simulink model "demd_dcMotor_separatelyExcit_f1"  (R2021a)
settings: Solver=VariableStepAuto  StartTime=0.0  StopTime=800  RelTol=1e-3
values from neighbouring files (symbols this model uses):
  B = (p_acc/3)/omega_n^2    (= 0.976675486798)    [demd_e2_dcMotor_separatelyExcited.m]
  C1 = 16.7/314    (= 0.0531847133758)    [demd_e2_dcMotor_separatelyExcited.m]
  C3 = 314/60    (= 5.23333333333)    [demd_e2_dcMotor_separatelyExcited.m]
  En = Ve/Ie    (= 120)    [demd_e2_dcMotor_separatelyExcited.m]
  Ie = 1    [demd_e2_dcMotor_separatelyExcited.m]
  J = M*v_max^2/omega_n^2    (= 73.2506615098)    [demd_e2_dcMotor_separatelyExcited.m]
  K = T_n/(I_n*Ie)    (= 1.71974522293)    [demd_e2_dcMotor_separatelyExcited.m]
  ki_curr = wia*Ra    (= 0.00168230769231)    [demd_e2_dcMotor_separatelyExcited.m]
  ki_exc = wie*Re    (= 24)    [demd_e2_dcMotor_separatelyExcited.m]
  ki_speed = ws*B    (= 1.9533509736)    [demd_e2_dcMotor_separatelyExcited.m]
  kp_curr = wia*La    (= 1.68230769231e-05)    [demd_e2_dcMotor_separatelyExcited.m]
  kp_exc = wie*Le    (= 24)    [demd_e2_dcMotor_separatelyExcited.m]
  kp_speed = ws*J    (= 146.50132302)    [demd_e2_dcMotor_separatelyExcited.m]
  La = Ra*tau_a    (= 0.000841153846154)    [demd_e2_dcMotor_separatelyExcited.m]
  Le = Re*tau_e    (= 120)    [demd_e2_dcMotor_separatelyExcited.m]
  Ra = (1-eta)*v_n/I_n    (= 0.0841153846154)    [demd_e2_dcMotor_separatelyExcited.m]
  Re = Ve/Ie    (= 120)    [demd_e2_dcMotor_separatelyExcited.m]
  T_n = p_tot/omega_n    (= 1226.70441142)    [demd_e2_dcMotor_separatelyExcited.m]
  v_n = 600    [demd_e2_dcMotor_separatelyExcited.m]
  Ve = 120    [demd_e2_dcMotor_separatelyExcited.m]
undefined symbols (not defined in the file or in its folder): Antiwindup
libraries: pid_lib x5, simulink x4
settings Model: Creator=mluser  LastModifiedBy=mluser
settings SolverCC: ZeroCrossAlgorithm=Adaptive  AlgebraicLoopSolver=TrustRegion
settings DebuggingCC: IgnoredZcDiagnostic=none

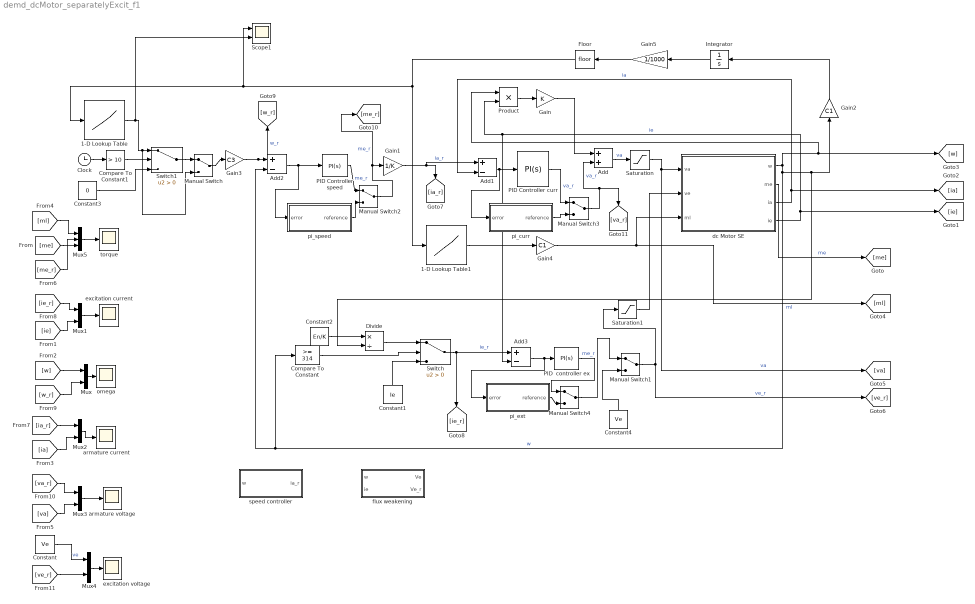
== system demd_dcMotor_separatelyExcit_f1 ==
  1-D Lookup Table : Lookup_n-D  NumberOfTableDimensions=1  BreakpointsForDimension1=[0 1 3 4 6 8 9 10]  Table=[35 60 60 75 60 60 35 0]  InterpMethod=Flat  InternalRulePriority=Speed  RndMeth=Simplest  InputSameDT=on
  1-D Lookup Table1 : Lookup_n-D  NumberOfTableDimensions=1  BreakpointsForDimension1=[0 1 3 4 6 8 9 10]  Table=[0 0 26000*9.81*sin(atan(5/100)) 0 0 26000*9.81*sin(atan(-5/100)) 0 0]  InterpMethod=Flat  InternalRulePriority=Speed  RndMeth=Simplest  InputSameDT=on
  Add : Sum
  Add1 : Sum  Inputs=+-
  Add2 : Sum  Inputs=+-
  Add3 : Sum  Inputs=+-
  Clock : Clock
  Compare To Constant : simulink/Logic and Bit Operations/Compare To Constant  relop=>=  const=314  OutDataTypeStr=boolean
  Compare To Constant1 : simulink/Logic and Bit Operations/Compare To Constant  relop=>  const=10  OutDataTypeStr=boolean
  Constant : Constant  Value=Ve
  Constant1 : Constant  Value=Ie
  Constant2 : Constant  Value=En/K
  Constant3 : Constant  Value=0
  Constant4 : Constant  Value=Ve
  Divide : Product  Inputs=*/
  Floor : Rounding
  Gain : Gain  Gain=K
  Gain1 : Gain  Gain=1/K
  Gain2 : Gain  Gain=C1
  Gain3 : Gain  Gain=C3
  Gain4 : Gain  Gain=C1
  Gain5 : Gain  Gain=1/1000
  Integrator : Integrator
  Manual Switch{,1..4} (5 alike) : ManualSwitch
  Mux{,1..4} (5 alike) : Mux  Inputs=2
  Mux5 : Mux  Inputs=3
  PID  controller ex : pid_lib/PID Controller  Controller=PI  Form=Parallel  TimeDomain=Continuous-time  UseExternalTs=off  SampleTime=-1  IntegratorMethod=Forward Euler  FilterMethod=Forward Euler  ControllerParametersSource=internal  P=kp_exc  I=ki_exc  D=0  UseFilter=on  N=100  TunerSelectOption=Transfer Function Based (PID Tuner App)  InitialConditionSource=internal  InitialConditionForIntegrator=0  InitialConditionForFilter=0  DifferentiatorICPrevScaledInput=0  ExternalReset=none  TrackingMode=off  Kt=1  LimitOutput=on  SatLimitsSource=internal  UpperSaturationLimit=Ve+Ve*0.3  LowerSaturationLimit=-1.3*Ve  LinearizeAsGain=on  AntiWindupMode=clamping  Kb=1  POutMin=[]  POutMax=[]  IOutMin=[]  IOutMax=[]  DOutMin=[]  DOutMax=[]  NOutMin=[]  NOutMax=[]  SumOutMin=[]  SumOutMax=[]  SaturationOutMin=[]  SaturationOutMax=[]  PParamMin=[]  PParamMax=[]  IParamMin=[]  IParamMax=[]  DParamMin=[]  DParamMax=[]  NParamMin=[]  NParamMax=[]  KbParamMin=[]  KbParamMax=[]  KtParamMin=[]  KtParamMax=[]  KbOutMin=[]  KbOutMax=[]  KtOutMin=[]  KtOutMax=[]  IntegratorOutMin=[]  IntegratorOutMax=[]  FilterOutMin=[]  FilterOutMax=[]  SumI1OutMin=[]  SumI1OutMax=[]  SumI2OutMin=[]  SumI2OutMax=[]  SumI3OutMin=[]  SumI3OutMax=[]  SumI4OutMin=[]  SumI4OutMax=[]  SumDOutMin=[]  SumDOutMax=[]  DifferentiatorOutMin=[]  DifferentiatorOutMax=[]  FilterDiffOutCoefMin=[]  FilterDiffOutCoefMax=[]  ReciprocalOutMin=[]  ReciprocalOutMax=[]  SumDenOutMin=[]  SumDenOutMax=[]  SumNumOutMin=[]  SumNumOutMax=[]  DivideOutMin=[]  DivideOutMax=[]  UdiffTsProdOutMin=[]  UdiffTsProdOutMax=[]  NTsProdOutMin=[]  NTsProdOutMax=[]  UintegralTsProdOutMin=[]  UintegralTsProdOutMax=[]  UngainTsProdOutMin=[]  UngainTsProdOutMax=[]  IntegratorContinuousStateAttributes=''  IntegratorStateMustResolveToSignalObject=off  IntegratorRTWStateStorageClass=Auto  FilterContinuousStateAttributes=''  FilterStateMustResolveToSignalObject=off  FilterRTWStateStorageClass=Auto  ParallelPVariant=InternalParameters  IdealPVariant=Disabled  IVariant=InternalParameters  DVariant=Disabled  IntegratorVariant=Continuous  SatVariant=Enabled  AWVariant=ContClampingParallel  PCopyVariant=Disabled  TRVariant=Disabled  FdbkBlocksVariant=Forward  IdealPFdbkVariant=Disabled  SatFdbkVariant=Disabled  DerivativeFilterVariant=Disabled  NVariant=Disabled  NCopyVariant=Disabled_SignalSpec  FilterICVariant=Disabled  IntegratorICVariant=InternalICs  ExternalResetVariant=Disabled  TRSumVariant=Passthrough  SumFdbkVariant=Disabled  SumVariant=Sum_PI  TsampFilterVariant=InternalTs  TsampNgainVariant=Passthrough  TsampIntegralVariant=Passthrough  ExternalSaturationOutDataTypeStr=Inherit: Same as second input
  PID Controller curr : pid_lib/PID Controller  Controller=PI  Form=Parallel  TimeDomain=Continuous-time  UseExternalTs=off  SampleTime=-1  IntegratorMethod=Forward Euler  FilterMethod=Forward Euler  ControllerParametersSource=internal  P=kp_curr  I=ki_curr  D=0  UseFilter=on  N=100  TunerSelectOption=Transfer Function Based (PID Tuner App)  InitialConditionSource=internal  InitialConditionForIntegrator=0  InitialConditionForFilter=0  DifferentiatorICPrevScaledInput=0  ExternalReset=none  TrackingMode=off  Kt=1  LimitOutput=on  SatLimitsSource=internal  UpperSaturationLimit=v_n+v_n*0.5  LowerSaturationLimit=-(v_n+v_n*0.5)  LinearizeAsGain=on  AntiWindupMode=clamping  Kb=1  POutMin=[]  POutMax=[]  IOutMin=[]  IOutMax=[]  DOutMin=[]  DOutMax=[]  NOutMin=[]  NOutMax=[]  SumOutMin=[]  SumOutMax=[]  SaturationOutMin=[]  SaturationOutMax=[]  PParamMin=[]  PParamMax=[]  IParamMin=[]  IParamMax=[]  DParamMin=[]  DParamMax=[]  NParamMin=[]  NParamMax=[]  KbParamMin=[]  KbParamMax=[]  KtParamMin=[]  KtParamMax=[]  KbOutMin=[]  KbOutMax=[]  KtOutMin=[]  KtOutMax=[]  IntegratorOutMin=[]  IntegratorOutMax=[]  FilterOutMin=[]  FilterOutMax=[]  SumI1OutMin=[]  SumI1OutMax=[]  SumI2OutMin=[]  SumI2OutMax=[]  SumI3OutMin=[]  SumI3OutMax=[]  SumI4OutMin=[]  SumI4OutMax=[]  SumDOutMin=[]  SumDOutMax=[]  DifferentiatorOutMin=[]  DifferentiatorOutMax=[]  FilterDiffOutCoefMin=[]  FilterDiffOutCoefMax=[]  ReciprocalOutMin=[]  ReciprocalOutMax=[]  SumDenOutMin=[]  SumDenOutMax=[]  SumNumOutMin=[]  SumNumOutMax=[]  DivideOutMin=[]  DivideOutMax=[]  UdiffTsProdOutMin=[]  UdiffTsProdOutMax=[]  NTsProdOutMin=[]  NTsProdOutMax=[]  UintegralTsProdOutMin=[]  UintegralTsProdOutMax=[]  UngainTsProdOutMin=[]  UngainTsProdOutMax=[]  IntegratorContinuousStateAttributes=''  IntegratorStateMustResolveToSignalObject=off  IntegratorRTWStateStorageClass=Auto  FilterContinuousStateAttributes=''  FilterStateMustResolveToSignalObject=off  FilterRTWStateStorageClass=Auto  ParallelPVariant=InternalParameters  IdealPVariant=Disabled  IVariant=InternalParameters  DVariant=Disabled  IntegratorVariant=Continuous  SatVariant=Enabled  AWVariant=ContClampingParallel  PCopyVariant=Disabled  TRVariant=Disabled  FdbkBlocksVariant=Forward  IdealPFdbkVariant=Disabled  SatFdbkVariant=Disabled  DerivativeFilterVariant=Disabled  NVariant=Disabled  NCopyVariant=Disabled_SignalSpec  FilterICVariant=Disabled  IntegratorICVariant=InternalICs  ExternalResetVariant=Disabled  TRSumVariant=Passthrough  SumFdbkVariant=Disabled  SumVariant=Sum_PI  TsampFilterVariant=InternalTs  TsampNgainVariant=Passthrough  TsampIntegralVariant=Passthrough  ExternalSaturationOutDataTypeStr=Inherit: Same as second input
  PID Controller speed : pid_lib/PID Controller  Controller=PI  Form=Parallel  TimeDomain=Continuous-time  UseExternalTs=off  SampleTime=-1  IntegratorMethod=Forward Euler  FilterMethod=Forward Euler  ControllerParametersSource=internal  P=kp_speed  I=ki_speed  D=0  UseFilter=on  N=100  TunerSelectOption=Transfer Function Based (PID Tuner App)  InitialConditionSource=internal  InitialConditionForIntegrator=0  InitialConditionForFilter=0  DifferentiatorICPrevScaledInput=0  ExternalReset=none  TrackingMode=off  Kt=1  LimitOutput=on  SatLimitsSource=internal  UpperSaturationLimit=1.5*T_n  LowerSaturationLimit=-1.5*T_n  LinearizeAsGain=on  AntiWindupMode=clamping  Kb=1  POutMin=[]  POutMax=[]  IOutMin=[]  IOutMax=[]  DOutMin=[]  DOutMax=[]  NOutMin=[]  NOutMax=[]  SumOutMin=[]  SumOutMax=[]  SaturationOutMin=[]  SaturationOutMax=[]  PParamMin=[]  PParamMax=[]  IParamMin=[]  IParamMax=[]  DParamMin=[]  DParamMax=[]  NParamMin=[]  NParamMax=[]  KbParamMin=[]  KbParamMax=[]  KtParamMin=[]  KtParamMax=[]  KbOutMin=[]  KbOutMax=[]  KtOutMin=[]  KtOutMax=[]  IntegratorOutMin=[]  IntegratorOutMax=[]  FilterOutMin=[]  FilterOutMax=[]  SumI1OutMin=[]  SumI1OutMax=[]  SumI2OutMin=[]  SumI2OutMax=[]  SumI3OutMin=[]  SumI3OutMax=[]  SumI4OutMin=[]  SumI4OutMax=[]  SumDOutMin=[]  SumDOutMax=[]  DifferentiatorOutMin=[]  DifferentiatorOutMax=[]  FilterDiffOutCoefMin=[]  FilterDiffOutCoefMax=[]  ReciprocalOutMin=[]  ReciprocalOutMax=[]  SumDenOutMin=[]  SumDenOutMax=[]  SumNumOutMin=[]  SumNumOutMax=[]  DivideOutMin=[]  DivideOutMax=[]  UdiffTsProdOutMin=[]  UdiffTsProdOutMax=[]  NTsProdOutMin=[]  NTsProdOutMax=[]  UintegralTsProdOutMin=[]  UintegralTsProdOutMax=[]  UngainTsProdOutMin=[]  UngainTsProdOutMax=[]  IntegratorContinuousStateAttributes=''  IntegratorStateMustResolveToSignalObject=off  IntegratorRTWStateStorageClass=Auto  FilterContinuousStateAttributes=''  FilterStateMustResolveToSignalObject=off  FilterRTWStateStorageClass=Auto  ParallelPVariant=InternalParameters  IdealPVariant=Disabled  IVariant=InternalParameters  DVariant=Disabled  IntegratorVariant=Continuous  SatVariant=Enabled  AWVariant=ContClampingParallel  PCopyVariant=Disabled  TRVariant=Disabled  FdbkBlocksVariant=Forward  IdealPFdbkVariant=Disabled  SatFdbkVariant=Disabled  DerivativeFilterVariant=Disabled  NVariant=Disabled  NCopyVariant=Disabled_SignalSpec  FilterICVariant=Disabled  IntegratorICVariant=InternalICs  ExternalResetVariant=Disabled  TRSumVariant=Passthrough  SumFdbkVariant=Disabled  SumVariant=Sum_PI  TsampFilterVariant=InternalTs  TsampNgainVariant=Passthrough  TsampIntegralVariant=Passthrough  ExternalSaturationOutDataTypeStr=Inherit: Same as second input
  Product : Product
  Saturation : Saturate  UpperLimit=v_n+v_n*0.5  LowerLimit=-(v_n+v_n*0.5)
  Saturation1 : Saturate  UpperLimit=Ve+0.3*Ve  LowerLimit=-Ve-0.3*Ve
  Scope1 : Scope  NumInputPorts=2
  Switch : Switch  Criteria=u2 > Threshold
  Switch1 : Switch  Criteria=u2 > Threshold
  armature current : Scope
  armature voltage : Scope
  dc Motor SE : Subsystem
  excitation current : Scope
  excitation voltage : Scope
  flux weakening : Subsystem
  omega : Scope
  pi_curr : Subsystem
  pi_ext : Subsystem
  pi_speed : Subsystem
  speed controller : Subsystem
  torque : Scope
  wires:
  PID Controller curr/1 -> Manual Switch3/1  "va_r"
  Add/1 -> Saturation/1  "va"
  dc Motor SE/3(ia) -> Add1/2, [ia]  "ia"
  Add1/1 -> pi_curr/1(error), PID Controller curr/1
  Gain1/1 -> [ia_r], Add1/1  "ia_r"
  PID Controller speed/1 -> Manual Switch2/1  "me_r"
  dc Motor SE/1(w) -> Product/1, [w], Compare To Constant/1, Add2/2, Divide/2, Gain2/1  "w"
  Add2/1 -> pi_speed/1(error), PID Controller speed/1
  Product/1 -> Gain/1
  dc Motor SE/4(ie) -> Add3/2, Product/2, [ie]  "ie"
  Gain2/1 -> Integrator/1
  Integrator/1 -> Gain5/1
  Floor/1 -> 1-D Lookup Table1/1, Scope1/1, 1-D Lookup Table/1
  Gain3/1 -> [w_r], Add2/1  "w_r"
  1-D Lookup Table1/1 -> Gain4/1
  Gain4/1 -> dc Motor SE/3(ml), [ml]  "ml"
  Add3/1 -> pi_ext/1(error), PID  controller ex/1
  Switch/1 -> Add3/1, [ie_r]  "ie_r"
  Constant1/1 -> Switch/3
  Constant2/1 -> Divide/1
  Divide/1 -> Switch/1
  Compare To Constant/1 -> Switch/2
  dc Motor SE/2(me) -> [me]  "me"
  [ie_r] -> Mux1/1
  [va_r] -> Mux3/1
  [ml] -> Mux5/1
  [me] -> Mux5/3
  [ie] -> Mux1/2
  [w_r] -> Mux/2
  [w] -> Mux/1
  Mux/1 -> omega/1
  Mux1/1 -> excitation current/1
  Constant/1 -> Mux4/1  "ve"
  [ve_r] -> Mux4/2
  Mux4/1 -> excitation voltage/1
  [ia_r] -> Mux2/1
  [ia] -> Mux2/2
  Mux2/1 -> armature current/1
  Mux3/1 -> armature voltage/1
  [va] -> Mux3/2
  [me_r] -> Mux5/2
  Mux5/1 -> torque/1
  1-D Lookup Table/1 -> Scope1/2, Manual Switch/2, Switch1/1
  Gain5/1 -> Floor/1
  Clock/1 -> Compare To Constant1/1
  Compare To Constant1/1 -> Switch1/2
  Constant3/1 -> Switch1/3
  Switch1/1 -> Manual Switch/1
  Manual Switch/1 -> Gain3/1
  Gain/1 -> Add/1
  Manual Switch1/1 -> [ve_r], Saturation1/1  "ve_r"
  PID  controller ex/1 -> Manual Switch4/1
  Constant4/1 -> Manual Switch1/2
  Manual Switch2/1 -> [me_r], Gain1/1  "me_r"
  pi_speed/1(reference) -> Manual Switch2/2
  pi_curr/1(reference) -> Manual Switch3/2
  Manual Switch3/1 -> Add/2, [va_r]  "va_r"
  pi_ext/1(reference) -> Manual Switch4/2
  Manual Switch4/1 -> Manual Switch1/1  "me_r"
  Saturation/1 -> [va], dc Motor SE/1(va)  "va"
  Saturation1/1 -> dc Motor SE/2(ve)

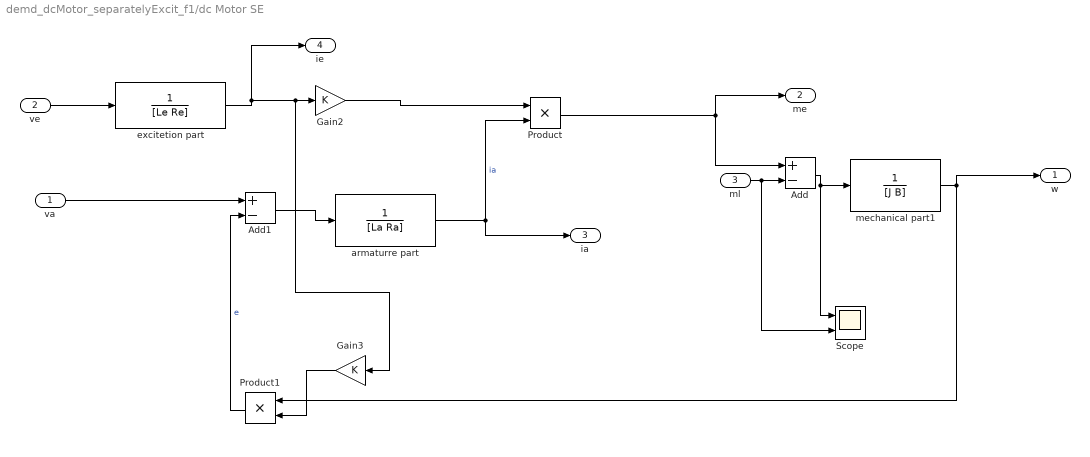
== system demd_dcMotor_separatelyExcit_f1/dc Motor SE ==
  va : Inport
  ve : Inport  Port=2
  ml : Inport  Port=3
  Add : Sum  Inputs=+-
  Add1 : Sum  Inputs=+-
  Gain2 : Gain  Gain=K
  Gain3 : Gain  Gain=K
  Product : Product
  Product1 : Product
  Scope : Scope  NumInputPorts=2
  armaturre part : TransferFcn  Denominator=[La Ra]
  excitetion part : TransferFcn  Denominator=[Le Re]
  mechanical part1 : TransferFcn  Denominator=[J B]
  w : Outport
  me : Outport  Port=2
  ia : Outport  Port=3
  ie : Outport  Port=4
  wires:
  mechanical part1/1 -> w/1, Product1/1
  Add/1 -> Scope/1, mechanical part1/1
  Product1/1 -> Add1/2  "e"
  va/1 -> Add1/1
  Add1/1 -> armaturre part/1
  armaturre part/1 -> Product/2, ia/1  "ia"
  Gain2/1 -> Product/1
  Product/1 -> Add/1, me/1
  ve/1 -> excitetion part/1
  excitetion part/1 -> ie/1, Gain3/1, Gain2/1
  Gain3/1 -> Product1/2
  ml/1 -> Scope/2, Add/2

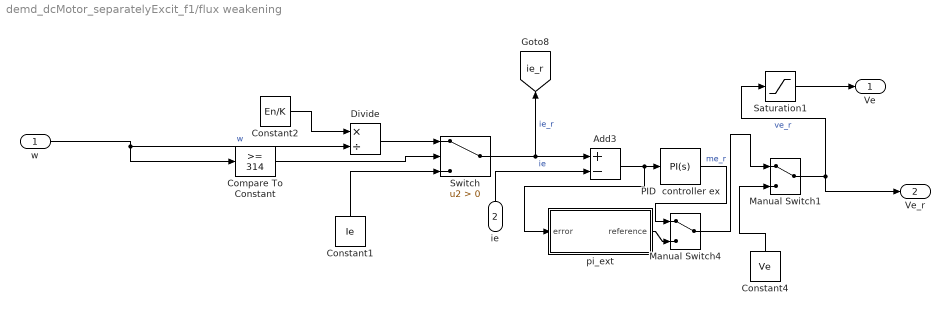
== system demd_dcMotor_separatelyExcit_f1/flux weakening ==
  w : Inport
  ie : Inport  Port=2
  Add3 : Sum  Inputs=+-
  Compare To Constant : simulink/Logic and Bit Operations/Compare To Constant  relop=>=  const=314  OutDataTypeStr=boolean
  Constant1 : Constant  Value=Ie
  Constant2 : Constant  Value=En/K
  Constant4 : Constant  Value=Ve
  Divide : Product  Inputs=*/
  Manual Switch1 : ManualSwitch
  Manual Switch4 : ManualSwitch
  PID  controller ex : pid_lib/PID Controller  Controller=PI  Form=Parallel  TimeDomain=Continuous-time  UseExternalTs=off  SampleTime=-1  IntegratorMethod=Forward Euler  FilterMethod=Forward Euler  ControllerParametersSource=internal  P=kp_exc  I=ki_exc  D=0  UseFilter=on  N=100  TunerSelectOption=Transfer Function Based (PID Tuner App)  InitialConditionSource=internal  InitialConditionForIntegrator=0  InitialConditionForFilter=0  DifferentiatorICPrevScaledInput=0  ExternalReset=none  TrackingMode=off  Kt=1  LimitOutput=on  SatLimitsSource=internal  UpperSaturationLimit=Ve+Ve*0.3  LowerSaturationLimit=-1.3*Ve  LinearizeAsGain=on  AntiWindupMode=clamping  Kb=1  POutMin=[]  POutMax=[]  IOutMin=[]  IOutMax=[]  DOutMin=[]  DOutMax=[]  NOutMin=[]  NOutMax=[]  SumOutMin=[]  SumOutMax=[]  SaturationOutMin=[]  SaturationOutMax=[]  PParamMin=[]  PParamMax=[]  IParamMin=[]  IParamMax=[]  DParamMin=[]  DParamMax=[]  NParamMin=[]  NParamMax=[]  KbParamMin=[]  KbParamMax=[]  KtParamMin=[]  KtParamMax=[]  KbOutMin=[]  KbOutMax=[]  KtOutMin=[]  KtOutMax=[]  IntegratorOutMin=[]  IntegratorOutMax=[]  FilterOutMin=[]  FilterOutMax=[]  SumI1OutMin=[]  SumI1OutMax=[]  SumI2OutMin=[]  SumI2OutMax=[]  SumI3OutMin=[]  SumI3OutMax=[]  SumI4OutMin=[]  SumI4OutMax=[]  SumDOutMin=[]  SumDOutMax=[]  DifferentiatorOutMin=[]  DifferentiatorOutMax=[]  FilterDiffOutCoefMin=[]  FilterDiffOutCoefMax=[]  ReciprocalOutMin=[]  ReciprocalOutMax=[]  SumDenOutMin=[]  SumDenOutMax=[]  SumNumOutMin=[]  SumNumOutMax=[]  DivideOutMin=[]  DivideOutMax=[]  UdiffTsProdOutMin=[]  UdiffTsProdOutMax=[]  NTsProdOutMin=[]  NTsProdOutMax=[]  UintegralTsProdOutMin=[]  UintegralTsProdOutMax=[]  UngainTsProdOutMin=[]  UngainTsProdOutMax=[]  IntegratorContinuousStateAttributes=''  IntegratorStateMustResolveToSignalObject=off  IntegratorRTWStateStorageClass=Auto  FilterContinuousStateAttributes=''  FilterStateMustResolveToSignalObject=off  FilterRTWStateStorageClass=Auto  ParallelPVariant=InternalParameters  IdealPVariant=Disabled  IVariant=InternalParameters  DVariant=Disabled  IntegratorVariant=Continuous  SatVariant=Enabled  AWVariant=ContClampingParallel  PCopyVariant=Disabled  TRVariant=Disabled  FdbkBlocksVariant=Forward  IdealPFdbkVariant=Disabled  SatFdbkVariant=Disabled  DerivativeFilterVariant=Disabled  NVariant=Disabled  NCopyVariant=Disabled_SignalSpec  FilterICVariant=Disabled  IntegratorICVariant=InternalICs  ExternalResetVariant=Disabled  TRSumVariant=Passthrough  SumFdbkVariant=Disabled  SumVariant=Sum_PI  TsampFilterVariant=InternalTs  TsampNgainVariant=Passthrough  TsampIntegralVariant=Passthrough  ExternalSaturationOutDataTypeStr=Inherit: Same as second input
  Saturation1 : Saturate  UpperLimit=Ve+0.3*Ve  LowerLimit=-Ve-0.3*Ve
  Switch : Switch  Criteria=u2 > Threshold
  pi_ext : Subsystem
  Ve : Outport
  Ve_r : Outport  Port=2
  tag scope: ie_r=global
  wires:
  PID  controller ex/1 -> Manual Switch4/1
  Constant2/1 -> Divide/1
  Manual Switch1/1 -> Ve_r/1, Saturation1/1  "ve_r"
  w/1 -> Divide/2, Compare To Constant/1  "w"
  Compare To Constant/1 -> Switch/2
  Saturation1/1 -> Ve/1
  Constant4/1 -> Manual Switch1/2
  Constant1/1 -> Switch/3
  Divide/1 -> Switch/1
  ie/1 -> Add3/2  "ie"
  Add3/1 -> pi_ext/1(error), PID  controller ex/1
  Switch/1 -> Add3/1, [ie_r]  "ie_r"
  Manual Switch4/1 -> Manual Switch1/1  "me_r"
  pi_ext/1(reference) -> Manual Switch4/2

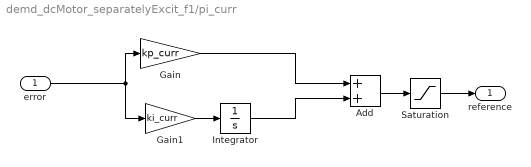
== system demd_dcMotor_separatelyExcit_f1/pi_curr ==
  error : Inport
  Add : Sum
  Gain : Gain  Gain=kp_curr
  Gain1 : Gain  Gain=ki_curr
  Integrator : Integrator
  Saturation : Saturate  UpperLimit=v_n+v_n*0.5  LowerLimit=-(v_n+v_n*0.5)
  reference : Outport
  wires:
  Gain/1 -> Add/1
  Gain1/1 -> Integrator/1
  Integrator/1 -> Add/2
  error/1 -> Gain/1, Gain1/1
  Add/1 -> Saturation/1
  Saturation/1 -> reference/1

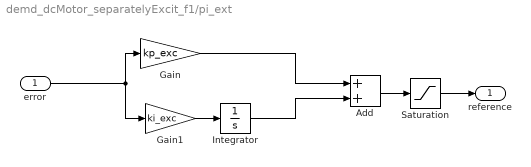
== system demd_dcMotor_separatelyExcit_f1/pi_ext ==
  error : Inport
  Add : Sum
  Gain : Gain  Gain=kp_exc
  Gain1 : Gain  Gain=ki_exc
  Integrator : Integrator
  Saturation : Saturate  UpperLimit=Ve+Ve*0.3  LowerLimit=-(Ve+Ve*0.3)
  reference : Outport
  wires:
  Gain/1 -> Add/1
  Gain1/1 -> Integrator/1
  Integrator/1 -> Add/2
  error/1 -> Gain/1, Gain1/1
  Add/1 -> Saturation/1
  Saturation/1 -> reference/1

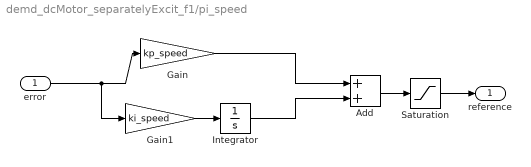
== system demd_dcMotor_separatelyExcit_f1/pi_speed ==
  error : Inport
  Add : Sum
  Gain : Gain  Gain=kp_speed
  Gain1 : Gain  Gain=ki_speed
  Integrator : Integrator  UpperSaturationLimit=Antiwindup  LowerSaturationLimit=-Antiwindup
  Saturation : Saturate  UpperLimit=1.5*T_n  LowerLimit=-(1.5*T_n)
  reference : Outport
  wires:
  Gain/1 -> Add/1
  Gain1/1 -> Integrator/1
  Integrator/1 -> Add/2
  error/1 -> Gain/1, Gain1/1
  Add/1 -> Saturation/1
  Saturation/1 -> reference/1

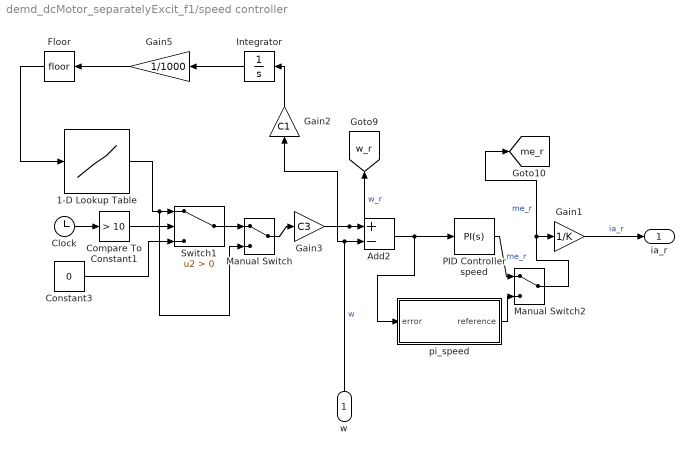
== system demd_dcMotor_separatelyExcit_f1/speed controller ==
  w : Inport
  1-D Lookup Table : Lookup_n-D  NumberOfTableDimensions=1  BreakpointsForDimension1=[0 1 3 4 6 8 9 10]  Table=[35 60 60 75 60 60 35 0]  InterpMethod=Flat  InternalRulePriority=Speed  RndMeth=Simplest  InputSameDT=on
  Add2 : Sum  Inputs=+-
  Clock : Clock
  Compare To Constant1 : simulink/Logic and Bit Operations/Compare To Constant  relop=>  const=10  OutDataTypeStr=boolean
  Constant3 : Constant  Value=0
  Floor : Rounding
  Gain1 : Gain  Gain=1/K
  Gain2 : Gain  Gain=C1
  Gain3 : Gain  Gain=C3
  Gain5 : Gain  Gain=1/1000
  Integrator : Integrator
  Manual Switch : ManualSwitch
  Manual Switch2 : ManualSwitch
  PID Controller speed : pid_lib/PID Controller  Controller=PI  Form=Parallel  TimeDomain=Continuous-time  UseExternalTs=off  SampleTime=-1  IntegratorMethod=Forward Euler  FilterMethod=Forward Euler  ControllerParametersSource=internal  P=kp_speed  I=ki_speed  D=0  UseFilter=on  N=100  TunerSelectOption=Transfer Function Based (PID Tuner App)  InitialConditionSource=internal  InitialConditionForIntegrator=0  InitialConditionForFilter=0  DifferentiatorICPrevScaledInput=0  ExternalReset=none  TrackingMode=off  Kt=1  LimitOutput=on  SatLimitsSource=internal  UpperSaturationLimit=1.5*T_n  LowerSaturationLimit=-1.5*T_n  LinearizeAsGain=on  AntiWindupMode=clamping  Kb=1  POutMin=[]  POutMax=[]  IOutMin=[]  IOutMax=[]  DOutMin=[]  DOutMax=[]  NOutMin=[]  NOutMax=[]  SumOutMin=[]  SumOutMax=[]  SaturationOutMin=[]  SaturationOutMax=[]  PParamMin=[]  PParamMax=[]  IParamMin=[]  IParamMax=[]  DParamMin=[]  DParamMax=[]  NParamMin=[]  NParamMax=[]  KbParamMin=[]  KbParamMax=[]  KtParamMin=[]  KtParamMax=[]  KbOutMin=[]  KbOutMax=[]  KtOutMin=[]  KtOutMax=[]  IntegratorOutMin=[]  IntegratorOutMax=[]  FilterOutMin=[]  FilterOutMax=[]  SumI1OutMin=[]  SumI1OutMax=[]  SumI2OutMin=[]  SumI2OutMax=[]  SumI3OutMin=[]  SumI3OutMax=[]  SumI4OutMin=[]  SumI4OutMax=[]  SumDOutMin=[]  SumDOutMax=[]  DifferentiatorOutMin=[]  DifferentiatorOutMax=[]  FilterDiffOutCoefMin=[]  FilterDiffOutCoefMax=[]  ReciprocalOutMin=[]  ReciprocalOutMax=[]  SumDenOutMin=[]  SumDenOutMax=[]  SumNumOutMin=[]  SumNumOutMax=[]  DivideOutMin=[]  DivideOutMax=[]  UdiffTsProdOutMin=[]  UdiffTsProdOutMax=[]  NTsProdOutMin=[]  NTsProdOutMax=[]  UintegralTsProdOutMin=[]  UintegralTsProdOutMax=[]  UngainTsProdOutMin=[]  UngainTsProdOutMax=[]  IntegratorContinuousStateAttributes=''  IntegratorStateMustResolveToSignalObject=off  IntegratorRTWStateStorageClass=Auto  FilterContinuousStateAttributes=''  FilterStateMustResolveToSignalObject=off  FilterRTWStateStorageClass=Auto  ParallelPVariant=InternalParameters  IdealPVariant=Disabled  IVariant=InternalParameters  DVariant=Disabled  IntegratorVariant=Continuous  SatVariant=Enabled  AWVariant=ContClampingParallel  PCopyVariant=Disabled  TRVariant=Disabled  FdbkBlocksVariant=Forward  IdealPFdbkVariant=Disabled  SatFdbkVariant=Disabled  DerivativeFilterVariant=Disabled  NVariant=Disabled  NCopyVariant=Disabled_SignalSpec  FilterICVariant=Disabled  IntegratorICVariant=InternalICs  ExternalResetVariant=Disabled  TRSumVariant=Passthrough  SumFdbkVariant=Disabled  SumVariant=Sum_PI  TsampFilterVariant=InternalTs  TsampNgainVariant=Passthrough  TsampIntegralVariant=Passthrough  ExternalSaturationOutDataTypeStr=Inherit: Same as second input
  Switch1 : Switch  Criteria=u2 > Threshold
  pi_speed : Subsystem
  ia_r : Outport
  tag scope: me_r=global, w_r=global
  wires:
  pi_speed/1(reference) -> Manual Switch2/2
  Constant3/1 -> Switch1/3
  Gain3/1 -> [w_r], Add2/1  "w_r"
  Add2/1 -> pi_speed/1(error), PID Controller speed/1
  PID Controller speed/1 -> Manual Switch2/1  "me_r"
  1-D Lookup Table/1 -> Manual Switch/2, Switch1/1
  Switch1/1 -> Manual Switch/1
  Gain1/1 -> ia_r/1  "ia_r"
  Compare To Constant1/1 -> Switch1/2
  Clock/1 -> Compare To Constant1/1
  w/1 -> Gain2/1, Add2/2  "w"
  Manual Switch/1 -> Gain3/1
  Manual Switch2/1 -> [me_r], Gain1/1  "me_r"
  Gain2/1 -> Integrator/1
  Integrator/1 -> Gain5/1
  Gain5/1 -> Floor/1
  Floor/1 -> 1-D Lookup Table/1

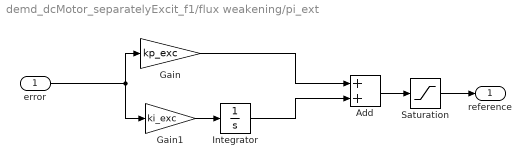
== system demd_dcMotor_separatelyExcit_f1/flux weakening/pi_ext ==
  error : Inport
  Add : Sum
  Gain : Gain  Gain=kp_exc
  Gain1 : Gain  Gain=ki_exc
  Integrator : Integrator
  Saturation : Saturate  UpperLimit=Ve+Ve*0.3  LowerLimit=-(Ve+Ve*0.3)
  reference : Outport
  wires:
  Gain/1 -> Add/1
  Gain1/1 -> Integrator/1
  Integrator/1 -> Add/2
  error/1 -> Gain/1, Gain1/1
  Add/1 -> Saturation/1
  Saturation/1 -> reference/1

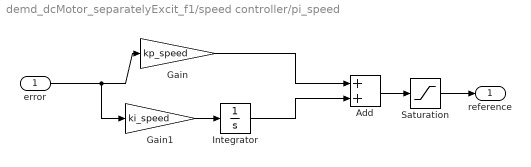
== system demd_dcMotor_separatelyExcit_f1/speed controller/pi_speed ==
  error : Inport
  Add : Sum
  Gain : Gain  Gain=kp_speed
  Gain1 : Gain  Gain=ki_speed
  Integrator : Integrator  UpperSaturationLimit=Antiwindup  LowerSaturationLimit=-Antiwindup
  Saturation : Saturate  UpperLimit=1.5*T_n  LowerLimit=-(1.5*T_n)
  reference : Outport
  wires:
  Gain/1 -> Add/1
  Gain1/1 -> Integrator/1
  Integrator/1 -> Add/2
  error/1 -> Gain/1, Gain1/1
  Add/1 -> Saturation/1
  Saturation/1 -> reference/1
